simulink model "copy_final"  (R2013a)
settings: Solver=ode45  StartTime=0.0  StopTime=150  RelTol=1e-3
model workspace (MAT data in the model file):
  i = 2
undefined symbols (not defined in the file): sigbuilder_block
(part 2 of 3)

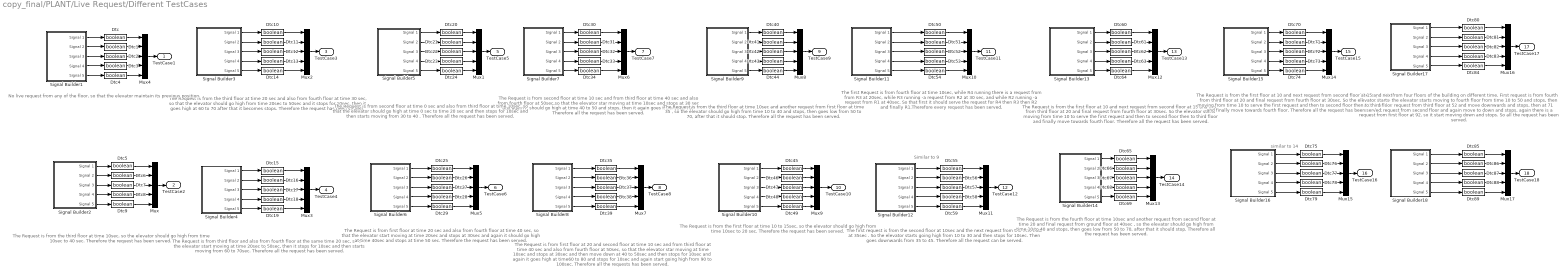
== system copy_final/PLANT/Live Request/Different TestCases ==
  note: The request is from four floors of the building on different time.
      |  First request is from fourth floor at 10, so the elevator  starts
      | moving to fourth floor from time 10 to 50 and stops, then at 50
      |  another request from third floor at 52 and move downwards
      |  and stops, then at 71 another request from second floor and
      | again move to down and stops, again there is a request from
      |  first floor at 92, so it start moving down
      | and stops. So all the request has been served.
  note: similar to 14
  note: Similar to 9
  note: The first request is from the second floor at 10sec and the next
      | request from the first floor at 35sec . So the elevator starts going
      | high from 10 to 30 and then stops for 10sec. Then goes downwards
      | from 35 to 45. Therefore all the request can be served.
  note: The Request is from third floor and also from fourth
      | floor at the same time 20 sec, so that the elevator
      | start moving at time 20sec to 50sec, then it stops
      |  for 10sec and then starts moving from 60 to 70sec.
      | Therefore all the request has been served.
  note: The Request is from the third floor at time 20 sec and
      | also from fourth floor at time 30 sec, so that the elevator
      | should go high from time 20sec to 50sec and it stops for
      | 10sec, then it goes high at 60 to 70 after that it becomes
      | stops. Therefore the request has been served.
  note: The Request is from first floor at time 20 sec and also
      |  from fourth floor at time 40 sec, so that the elevator start
      |  moving at time 20sec and stops at 30sec and again it
      | should go high at time 40sec and stops at time 50 sec.
      | Therefore the request has been served.
  note: The Request is from second floor at time 10 sec and from third
      |  floor at time 40 sec and also from fourth floor at 50sec,so that
      | the elevator star moving at time 10sec and stops at 30 sec and
      | again it should go high at time 40 to 50 and stops, then it again
      | goes from 60 to 70. Therefore all the request has been served.
  note: The Request is from first floor at 20 and second floor at time 10 sec
      |  and from third floor at time 40 sec and also from fourth floor at 50sec,
      | so that the elevator star moving at time 10sec and stops at 30sec
      | and then move down at 40 to 50sec and then stops for 10sec and
      | again it goes high at time60 to 80 and stops for 10sec and again
      |  start going high from 90 to 100sec. Therefore all the requests has
      |  been served.
  note: The Request is from the third floor at time 10sec and another
      | request from first floor at time 35 , so the elevator should go
      | high from time 10 to 40 and stops, then goes low from
      | 50 to 70, after that it should stop. Therefore all the
      |  request has been served.
  note: The Request is from the first floor at time 10 to 15sec,
      |  so the elevator should go high from time 10sec to
      | 20 sec. Therefore the request has been served.
  note: The first Request is from fourth floor at time 10sec, while R4 running there
      |  is a request from  from R3 at 20sec, while R3 running -a request from R2
      | at 30 sec, and while R2 running -a request from R1 at 40sec. So that first
      | it should serve the request for R4 then R3 then R2 and finally R1.Therefore
      |  every request has been served.
  note: The Request is from the first floor at 10 and next request from
      | second floor at 15 and next from third floor at 20 and final
      | request from fourth floor at 30sec. So the elevator starts
      | moving from time 10 to serve the first request and then to
      |  second floor  then to third floor and finally move towards
      | fourth floor. Therefore all the request has been served.
  note: No live request from any of the floor, so that
      | the elevator maintain its previous position.
  note: The Request is from the third floor at time 10sec,
      |  so the elevator should go high from time 10sec to
      | 40 sec. Therefore the request has been served.
  note: The Request is from second floor at time 0 sec and also
      |  from third floor at time 10sec, so that the elevator should
      | go high at time 0 sec  to time 20 sec and then stops for
      | 10sec and then starts moving from 30 to 40 . Therefore
      | all the request has been served.
  note: The Request is from the fourth floor at time 10sec and another
      | request from second floor at time 20 and final request from
      | ground floor at 40sec , so the elevator should go
      | high from time 10 to 40 and stops, then goes low from
      | 50 to 70, after that it should stop. Therefore all the
      |  request has been served.
  note: The Request is from the first floor at 10 and next request from
      | second floor at 15 and next from third floor at 20 and final
      | request from fourth floor at 30sec. So the elevator starts
      | moving from time 10 to serve the first request and then to
      |  second floor  then to third floor and finally move towards
      | fourth floor. Therefore all the request has been served.
  Dtc{,1..89} (90 alike) : DataTypeConversion  OutDataTypeStr=boolean
  Mux{,1..17} (18 alike) : Mux  Inputs=5
  Signal Builder1 : Subsystem  Tag=STV Subsys  LoadFcn=sigbuilder_block('load');  StartFcn=sigbuilder_block('start');  StopFcn=sigbuilder_block('stop');  ClipboardFcn=sigbuilder_block('clipboard');  mask(Sigbuilder block){}
      mask help: Simulink:masks:SigbuilderBlock_MD
      mask init:
      | if ~strcmp(get_param(bdroot(gcbh),'SimulationStatus'),'stopped') tuvar = sigbuilder_block('maskInit'); end
      settings: CopyFcn=sigbuilder_block('copy');  DeleteFcn=sigbuilder_block('delete');  ModelCloseFcn=sigbuilder_block('modelClose');  PreSaveFcn=sigbuilder_block('preSave');  PauseFcn=sigbuilder_block('pause');  ContinueFcn=sigbuilder_block('continue');  NameChangeFcn=sigbuilder_block('namechange');  OpenFcn=sigbuilder_block('open',[327.75 102.75 484.5 312.75 ]);  CloseFcn=sigbuilder_block('close');
      mask Display: plot(0, 0, 100, 100,[2, 2, 32, 32, 2], [68, 8, 8, 68, 68],[32, 2], [38, 38], [32, 19, 2],[53, 60, 44], [32, 17, 17, 2],[16, 16, 31, 31]);txt = getActiveGroup(gcbh);text(2, 100, txt,'verticalAlignment', 'top');
  Signal Builder10 : Subsystem  Tag=STV Subsys  LoadFcn=sigbuilder_block('load');  StartFcn=sigbuilder_block('start');  StopFcn=sigbuilder_block('stop');  ClipboardFcn=sigbuilder_block('clipboard');  mask(Sigbuilder block){}
      mask help: Simulink:masks:SigbuilderBlock_MD
      mask init:
      | if ~strcmp(get_param(bdroot(gcbh),'SimulationStatus'),'stopped') tuvar = sigbuilder_block('maskInit'); end
      settings: CopyFcn=sigbuilder_block('copy');  DeleteFcn=sigbuilder_block('delete');  ModelCloseFcn=sigbuilder_block('modelClose');  PreSaveFcn=sigbuilder_block('preSave');  PauseFcn=sigbuilder_block('pause');  ContinueFcn=sigbuilder_block('continue');  NameChangeFcn=sigbuilder_block('namechange');  OpenFcn=sigbuilder_block('open',[437.25 118.5 550.5 394.5 ]);  CloseFcn=sigbuilder_block('close');
      mask Display: plot(0, 0, 100, 100,[2, 2, 32, 32, 2], [68, 8, 8, 68, 68],[32, 2], [38, 38], [32, 19, 2],[53, 60, 44], [32, 17, 17, 2],[16, 16, 31, 31]);txt = getActiveGroup(gcbh);text(2, 100, txt,'verticalAlignment', 'top');
  Signal Builder11 : Subsystem  Tag=STV Subsys  LoadFcn=sigbuilder_block('load');  StartFcn=sigbuilder_block('start');  StopFcn=sigbuilder_block('stop');  ClipboardFcn=sigbuilder_block('clipboard');  mask(Sigbuilder block){}
      mask help: Simulink:masks:SigbuilderBlock_MD
      mask init:
      | if ~strcmp(get_param(bdroot(gcbh),'SimulationStatus'),'stopped') tuvar = sigbuilder_block('maskInit'); end
      settings: CopyFcn=sigbuilder_block('copy');  DeleteFcn=sigbuilder_block('delete');  ModelCloseFcn=sigbuilder_block('modelClose');  PreSaveFcn=sigbuilder_block('preSave');  PauseFcn=sigbuilder_block('pause');  ContinueFcn=sigbuilder_block('continue');  NameChangeFcn=sigbuilder_block('namechange');  OpenFcn=sigbuilder_block('open',[344.25 118.5 602.25 275.25 ]);  CloseFcn=sigbuilder_block('close');
      mask Display: plot(0, 0, 100, 100,[2, 2, 32, 32, 2], [68, 8, 8, 68, 68],[32, 2], [38, 38], [32, 19, 2],[53, 60, 44], [32, 17, 17, 2],[16, 16, 31, 31]);txt = getActiveGroup(gcbh);text(2, 100, txt,'verticalAlignment', 'top');
  Signal Builder12 : Subsystem  Tag=STV Subsys  LoadFcn=sigbuilder_block('load');  StartFcn=sigbuilder_block('start');  StopFcn=sigbuilder_block('stop');  ClipboardFcn=sigbuilder_block('clipboard');  mask(Sigbuilder block){}
      mask help: Simulink:masks:SigbuilderBlock_MD
      mask init:
      | if ~strcmp(get_param(bdroot(gcbh),'SimulationStatus'),'stopped') tuvar = sigbuilder_block('maskInit'); end
      settings: CopyFcn=sigbuilder_block('copy');  DeleteFcn=sigbuilder_block('delete');  ModelCloseFcn=sigbuilder_block('modelClose');  PreSaveFcn=sigbuilder_block('preSave');  PauseFcn=sigbuilder_block('pause');  ContinueFcn=sigbuilder_block('continue');  NameChangeFcn=sigbuilder_block('namechange');  OpenFcn=sigbuilder_block('open',[393.75 66.75 550.5 275.25 ]);  CloseFcn=sigbuilder_block('close');
      mask Display: plot(0, 0, 100, 100,[2, 2, 32, 32, 2], [68, 8, 8, 68, 68],[32, 2], [38, 38], [32, 19, 2],[53, 60, 44], [32, 17, 17, 2],[16, 16, 31, 31]);txt = getActiveGroup(gcbh);text(2, 100, txt,'verticalAlignment', 'top');
  Signal Builder13 : Subsystem  Tag=STV Subsys  LoadFcn=sigbuilder_block('load');  StartFcn=sigbuilder_block('start');  StopFcn=sigbuilder_block('stop');  ClipboardFcn=sigbuilder_block('clipboard');  mask(Sigbuilder block){}
      mask help: Simulink:masks:SigbuilderBlock_MD
      mask init:
      | if ~strcmp(get_param(bdroot(gcbh),'SimulationStatus'),'stopped') tuvar = sigbuilder_block('maskInit'); end
      settings: CopyFcn=sigbuilder_block('copy');  DeleteFcn=sigbuilder_block('delete');  ModelCloseFcn=sigbuilder_block('modelClose');  PreSaveFcn=sigbuilder_block('preSave');  PauseFcn=sigbuilder_block('pause');  ContinueFcn=sigbuilder_block('continue');  NameChangeFcn=sigbuilder_block('namechange');  OpenFcn=sigbuilder_block('open',[274.5 170.25 550.5 272.25 ]);  CloseFcn=sigbuilder_block('close');
      mask Display: plot(0, 0, 100, 100,[2, 2, 32, 32, 2], [68, 8, 8, 68, 68],[32, 2], [38, 38], [32, 19, 2],[53, 60, 44], [32, 17, 17, 2],[16, 16, 31, 31]);txt = getActiveGroup(gcbh);text(2, 100, txt,'verticalAlignment', 'top');
  Signal Builder14 : Subsystem  Tag=STV Subsys  LoadFcn=sigbuilder_block('load');  StartFcn=sigbuilder_block('start');  StopFcn=sigbuilder_block('stop');  ClipboardFcn=sigbuilder_block('clipboard');  mask(Sigbuilder block){}
      mask help: Simulink:masks:SigbuilderBlock_MD
      mask init:
      | if ~strcmp(get_param(bdroot(gcbh),'SimulationStatus'),'stopped') tuvar = sigbuilder_block('maskInit'); end
      settings: CopyFcn=sigbuilder_block('copy');  DeleteFcn=sigbuilder_block('delete');  ModelCloseFcn=sigbuilder_block('modelClose');  PreSaveFcn=sigbuilder_block('preSave');  PauseFcn=sigbuilder_block('pause');  ContinueFcn=sigbuilder_block('continue');  NameChangeFcn=sigbuilder_block('namechange');  OpenFcn=sigbuilder_block('open',[507.75 134.25 448.5 303.75 ]);  CloseFcn=sigbuilder_block('close');
      mask Display: plot(0, 0, 100, 100,[2, 2, 32, 32, 2], [68, 8, 8, 68, 68],[32, 2], [38, 38], [32, 19, 2],[53, 60, 44], [32, 17, 17, 2],[16, 16, 31, 31]);txt = getActiveGroup(gcbh);text(2, 100, txt,'verticalAlignment', 'top');
  Signal Builder15 : Subsystem  Tag=STV Subsys  LoadFcn=sigbuilder_block('load');  StartFcn=sigbuilder_block('start');  StopFcn=sigbuilder_block('stop');  ClipboardFcn=sigbuilder_block('clipboard');  mask(Sigbuilder block){}
      mask help: Simulink:masks:SigbuilderBlock_MD
      mask init:
      | if ~strcmp(get_param(bdroot(gcbh),'SimulationStatus'),'stopped') tuvar = sigbuilder_block('maskInit'); end
      settings: CopyFcn=sigbuilder_block('copy');  DeleteFcn=sigbuilder_block('delete');  ModelCloseFcn=sigbuilder_block('modelClose');  PreSaveFcn=sigbuilder_block('preSave');  PauseFcn=sigbuilder_block('pause');  ContinueFcn=sigbuilder_block('continue');  NameChangeFcn=sigbuilder_block('namechange');  OpenFcn=sigbuilder_block('open',[465.75 164.25 447 288.75 ]);  CloseFcn=sigbuilder_block('close');
      mask Display: plot(0, 0, 100, 100,[2, 2, 32, 32, 2], [68, 8, 8, 68, 68],[32, 2], [38, 38], [32, 19, 2],[53, 60, 44], [32, 17, 17, 2],[16, 16, 31, 31]);txt = getActiveGroup(gcbh);text(2, 100, txt,'verticalAlignment', 'top');
  Signal Builder16 : Subsystem  Tag=STV Subsys  LoadFcn=sigbuilder_block('load');  StartFcn=sigbuilder_block('start');  StopFcn=sigbuilder_block('stop');  ClipboardFcn=sigbuilder_block('clipboard');  mask(Sigbuilder block){}
      mask help: Simulink:masks:SigbuilderBlock_MD
      mask init:
      | if ~strcmp(get_param(bdroot(gcbh),'SimulationStatus'),'stopped') tuvar = sigbuilder_block('maskInit'); end
      settings: CopyFcn=sigbuilder_block('copy');  DeleteFcn=sigbuilder_block('delete');  ModelCloseFcn=sigbuilder_block('modelClose');  PreSaveFcn=sigbuilder_block('preSave');  PauseFcn=sigbuilder_block('pause');  ContinueFcn=sigbuilder_block('continue');  NameChangeFcn=sigbuilder_block('namechange');  OpenFcn=sigbuilder_block('open',[451.5 37.5 549 315.75 ]);  CloseFcn=sigbuilder_block('close');
      mask Display: plot(0, 0, 100, 100,[2, 2, 32, 32, 2], [68, 8, 8, 68, 68],[32, 2], [38, 38], [32, 19, 2],[53, 60, 44], [32, 17, 17, 2],[16, 16, 31, 31]);txt = getActiveGroup(gcbh);text(2, 100, txt,'verticalAlignment', 'top');
  Signal Builder17 : Subsystem  Tag=STV Subsys  LoadFcn=sigbuilder_block('load');  StartFcn=sigbuilder_block('start');  StopFcn=sigbuilder_block('stop');  ClipboardFcn=sigbuilder_block('clipboard');  mask(Sigbuilder block){}
      mask help: Simulink:masks:SigbuilderBlock_MD
      mask init:
      | if ~strcmp(get_param(bdroot(gcbh),'SimulationStatus'),'stopped') tuvar = sigbuilder_block('maskInit'); end
      settings: CopyFcn=sigbuilder_block('copy');  DeleteFcn=sigbuilder_block('delete');  ModelCloseFcn=sigbuilder_block('modelClose');  PreSaveFcn=sigbuilder_block('preSave');  PauseFcn=sigbuilder_block('pause');  ContinueFcn=sigbuilder_block('continue');  NameChangeFcn=sigbuilder_block('namechange');  OpenFcn=sigbuilder_block('open',[428.25 139.5 438.75 335.25 ]);  CloseFcn=sigbuilder_block('close');
      mask Display: plot(0, 0, 100, 100,[2, 2, 32, 32, 2], [68, 8, 8, 68, 68],[32, 2], [38, 38], [32, 19, 2],[53, 60, 44], [32, 17, 17, 2],[16, 16, 31, 31]);txt = getActiveGroup(gcbh);text(2, 100, txt,'verticalAlignment', 'top');
  Signal Builder18 : Subsystem  Tag=STV Subsys  LoadFcn=sigbuilder_block('load');  StartFcn=sigbuilder_block('start');  StopFcn=sigbuilder_block('stop');  ClipboardFcn=sigbuilder_block('clipboard');  mask(Sigbuilder block){}
      mask help: Simulink:masks:SigbuilderBlock_MD
      mask init:
      | if ~strcmp(get_param(bdroot(gcbh),'SimulationStatus'),'stopped') tuvar = sigbuilder_block('maskInit'); end
      settings: CopyFcn=sigbuilder_block('copy');  DeleteFcn=sigbuilder_block('delete');  ModelCloseFcn=sigbuilder_block('modelClose');  PreSaveFcn=sigbuilder_block('preSave');  PauseFcn=sigbuilder_block('pause');  ContinueFcn=sigbuilder_block('continue');  NameChangeFcn=sigbuilder_block('namechange');  OpenFcn=sigbuilder_block('open',[406.5 184.5 604.5 275.25 ]);  CloseFcn=sigbuilder_block('close');
      mask Display: plot(0, 0, 100, 100,[2, 2, 32, 32, 2], [68, 8, 8, 68, 68],[32, 2], [38, 38], [32, 19, 2],[53, 60, 44], [32, 17, 17, 2],[16, 16, 31, 31]);txt = getActiveGroup(gcbh);text(2, 100, txt,'verticalAlignment', 'top');
  Signal Builder2 : Subsystem  Tag=STV Subsys  LoadFcn=sigbuilder_block('load');  StartFcn=sigbuilder_block('start');  StopFcn=sigbuilder_block('stop');  ClipboardFcn=sigbuilder_block('clipboard');  mask(Sigbuilder block){}
      mask help: Simulink:masks:SigbuilderBlock_MD
      mask init:
      | if ~strcmp(get_param(bdroot(gcbh),'SimulationStatus'),'stopped') tuvar = sigbuilder_block('maskInit'); end
      settings: CopyFcn=sigbuilder_block('copy');  DeleteFcn=sigbuilder_block('delete');  ModelCloseFcn=sigbuilder_block('modelClose');  PreSaveFcn=sigbuilder_block('preSave');  PauseFcn=sigbuilder_block('pause');  ContinueFcn=sigbuilder_block('continue');  NameChangeFcn=sigbuilder_block('namechange');  OpenFcn=sigbuilder_block('open',[286.5 116.25 459.75 300.75 ]);  CloseFcn=sigbuilder_block('close');
      mask Display: plot(0, 0, 100, 100,[2, 2, 32, 32, 2], [68, 8, 8, 68, 68],[32, 2], [38, 38], [32, 19, 2],[53, 60, 44], [32, 17, 17, 2],[16, 16, 31, 31]);txt = getActiveGroup(gcbh);text(2, 100, txt,'verticalAlignment', 'top');
  Signal Builder3 : Subsystem  Tag=STV Subsys  LoadFcn=sigbuilder_block('load');  StartFcn=sigbuilder_block('start');  StopFcn=sigbuilder_block('stop');  ClipboardFcn=sigbuilder_block('clipboard');  mask(Sigbuilder block){}
      mask help: Simulink:masks:SigbuilderBlock_MD
      mask init:
      | if ~strcmp(get_param(bdroot(gcbh),'SimulationStatus'),'stopped') tuvar = sigbuilder_block('maskInit'); end
      settings: CopyFcn=sigbuilder_block('copy');  DeleteFcn=sigbuilder_block('delete');  ModelCloseFcn=sigbuilder_block('modelClose');  PreSaveFcn=sigbuilder_block('preSave');  PauseFcn=sigbuilder_block('pause');  ContinueFcn=sigbuilder_block('continue');  NameChangeFcn=sigbuilder_block('namechange');  OpenFcn=sigbuilder_block('open',[365.25 119.25 436.5 279 ]);  CloseFcn=sigbuilder_block('close');
      mask Display: plot(0, 0, 100, 100,[2, 2, 32, 32, 2], [68, 8, 8, 68, 68],[32, 2], [38, 38], [32, 19, 2],[53, 60, 44], [32, 17, 17, 2],[16, 16, 31, 31]);txt = getActiveGroup(gcbh);text(2, 100, txt,'verticalAlignment', 'top');
  Signal Builder4 : Subsystem  Tag=STV Subsys  LoadFcn=sigbuilder_block('load');  StartFcn=sigbuilder_block('start');  StopFcn=sigbuilder_block('stop');  ClipboardFcn=sigbuilder_block('clipboard');  mask(Sigbuilder block){}
      mask help: Simulink:masks:SigbuilderBlock_MD
      mask init:
      | if ~strcmp(get_param(bdroot(gcbh),'SimulationStatus'),'stopped') tuvar = sigbuilder_block('maskInit'); end
      settings: CopyFcn=sigbuilder_block('copy');  DeleteFcn=sigbuilder_block('delete');  ModelCloseFcn=sigbuilder_block('modelClose');  PreSaveFcn=sigbuilder_block('preSave');  PauseFcn=sigbuilder_block('pause');  ContinueFcn=sigbuilder_block('continue');  NameChangeFcn=sigbuilder_block('namechange');  OpenFcn=sigbuilder_block('open',[336.75 135.75 495 312.75 ]);  CloseFcn=sigbuilder_block('close');
      mask Display: plot(0, 0, 100, 100,[2, 2, 32, 32, 2], [68, 8, 8, 68, 68],[32, 2], [38, 38], [32, 19, 2],[53, 60, 44], [32, 17, 17, 2],[16, 16, 31, 31]);txt = getActiveGroup(gcbh);text(2, 100, txt,'verticalAlignment', 'top');
  Signal Builder5 : Subsystem  Tag=STV Subsys  LoadFcn=sigbuilder_block('load');  StartFcn=sigbuilder_block('start');  StopFcn=sigbuilder_block('stop');  ClipboardFcn=sigbuilder_block('clipboard');  mask(Sigbuilder block){}
      mask help: Simulink:masks:SigbuilderBlock_MD
      mask init:
      | if ~strcmp(get_param(bdroot(gcbh),'SimulationStatus'),'stopped') tuvar = sigbuilder_block('maskInit'); end
      settings: CopyFcn=sigbuilder_block('copy');  DeleteFcn=sigbuilder_block('delete');  ModelCloseFcn=sigbuilder_block('modelClose');  PreSaveFcn=sigbuilder_block('preSave');  PauseFcn=sigbuilder_block('pause');  ContinueFcn=sigbuilder_block('continue');  NameChangeFcn=sigbuilder_block('namechange');  OpenFcn=sigbuilder_block('open',[328.5 -1.5 550.5 394.5 ]);  CloseFcn=sigbuilder_block('close');
      mask Display: plot(0, 0, 100, 100,[2, 2, 32, 32, 2], [68, 8, 8, 68, 68],[32, 2], [38, 38], [32, 19, 2],[53, 60, 44], [32, 17, 17, 2],[16, 16, 31, 31]);txt = getActiveGroup(gcbh);text(2, 100, txt,'verticalAlignment', 'top');
  Signal Builder6 : Subsystem  Tag=STV Subsys  LoadFcn=sigbuilder_block('load');  StartFcn=sigbuilder_block('start');  StopFcn=sigbuilder_block('stop');  ClipboardFcn=sigbuilder_block('clipboard');  mask(Sigbuilder block){}
      mask help: Simulink:masks:SigbuilderBlock_MD
      mask init:
      | if ~strcmp(get_param(bdroot(gcbh),'SimulationStatus'),'stopped') tuvar = sigbuilder_block('maskInit'); end
      settings: CopyFcn=sigbuilder_block('copy');  DeleteFcn=sigbuilder_block('delete');  ModelCloseFcn=sigbuilder_block('modelClose');  PreSaveFcn=sigbuilder_block('preSave');  PauseFcn=sigbuilder_block('pause');  ContinueFcn=sigbuilder_block('continue');  NameChangeFcn=sigbuilder_block('namechange');  OpenFcn=sigbuilder_block('open',[91.5 55.5 550.5 394.5 ]);  CloseFcn=sigbuilder_block('close');
      mask Display: plot(0, 0, 100, 100,[2, 2, 32, 32, 2], [68, 8, 8, 68, 68],[32, 2], [38, 38], [32, 19, 2],[53, 60, 44], [32, 17, 17, 2],[16, 16, 31, 31]);txt = getActiveGroup(gcbh);text(2, 100, txt,'verticalAlignment', 'top');
  Signal Builder7 : Subsystem  Tag=STV Subsys  LoadFcn=sigbuilder_block('load');  StartFcn=sigbuilder_block('start');  StopFcn=sigbuilder_block('stop');  ClipboardFcn=sigbuilder_block('clipboard');  mask(Sigbuilder block){}
      mask help: Simulink:masks:SigbuilderBlock_MD
      mask init:
      | if ~strcmp(get_param(bdroot(gcbh),'SimulationStatus'),'stopped') tuvar = sigbuilder_block('maskInit'); end
      settings: CopyFcn=sigbuilder_block('copy');  DeleteFcn=sigbuilder_block('delete');  ModelCloseFcn=sigbuilder_block('modelClose');  PreSaveFcn=sigbuilder_block('preSave');  PauseFcn=sigbuilder_block('pause');  ContinueFcn=sigbuilder_block('continue');  NameChangeFcn=sigbuilder_block('namechange');  OpenFcn=sigbuilder_block('open',[87 91.5 512.25 357 ]);  CloseFcn=sigbuilder_block('close');
      mask Display: plot(0, 0, 100, 100,[2, 2, 32, 32, 2], [68, 8, 8, 68, 68],[32, 2], [38, 38], [32, 19, 2],[53, 60, 44], [32, 17, 17, 2],[16, 16, 31, 31]);txt = getActiveGroup(gcbh);text(2, 100, txt,'verticalAlignment', 'top');
  Signal Builder8 : Subsystem  Tag=STV Subsys  LoadFcn=sigbuilder_block('load');  StartFcn=sigbuilder_block('start');  StopFcn=sigbuilder_block('stop');  ClipboardFcn=sigbuilder_block('clipboard');  mask(Sigbuilder block){}
      mask help: Simulink:masks:SigbuilderBlock_MD
      mask init:
      | if ~strcmp(get_param(bdroot(gcbh),'SimulationStatus'),'stopped') tuvar = sigbuilder_block('maskInit'); end
      settings: CopyFcn=sigbuilder_block('copy');  DeleteFcn=sigbuilder_block('delete');  ModelCloseFcn=sigbuilder_block('modelClose');  PreSaveFcn=sigbuilder_block('preSave');  PauseFcn=sigbuilder_block('pause');  ContinueFcn=sigbuilder_block('continue');  NameChangeFcn=sigbuilder_block('namechange');  OpenFcn=sigbuilder_block('open',[269.25 168.75 480 285 ]);  CloseFcn=sigbuilder_block('close');
      mask Display: plot(0, 0, 100, 100,[2, 2, 32, 32, 2], [68, 8, 8, 68, 68],[32, 2], [38, 38], [32, 19, 2],[53, 60, 44], [32, 17, 17, 2],[16, 16, 31, 31]);txt = getActiveGroup(gcbh);text(2, 100, txt,'verticalAlignment', 'top');
  Signal Builder9 : Subsystem  Tag=STV Subsys  LoadFcn=sigbuilder_block('load');  StartFcn=sigbuilder_block('start');  StopFcn=sigbuilder_block('stop');  ClipboardFcn=sigbuilder_block('clipboard');  mask(Sigbuilder block){}
      mask help: Simulink:masks:SigbuilderBlock_MD
      mask init:
      | if ~strcmp(get_param(bdroot(gcbh),'SimulationStatus'),'stopped') tuvar = sigbuilder_block('maskInit'); end
      settings: CopyFcn=sigbuilder_block('copy');  DeleteFcn=sigbuilder_block('delete');  ModelCloseFcn=sigbuilder_block('modelClose');  PreSaveFcn=sigbuilder_block('preSave');  PauseFcn=sigbuilder_block('pause');  ContinueFcn=sigbuilder_block('continue');  NameChangeFcn=sigbuilder_block('namechange');  OpenFcn=sigbuilder_block('open',[549 141.75 414 282.75 ]);  CloseFcn=sigbuilder_block('close');
      mask Display: plot(0, 0, 100, 100,[2, 2, 32, 32, 2], [68, 8, 8, 68, 68],[32, 2], [38, 38], [32, 19, 2],[53, 60, 44], [32, 17, 17, 2],[16, 16, 31, 31]);txt = getActiveGroup(gcbh);text(2, 100, txt,'verticalAlignment', 'top');
  TestCase1 : Outport  OutDataTypeStr=boolean
  TestCase2 : Outport  Port=2  OutDataTypeStr=boolean
  TestCase3 : Outport  Port=3  OutDataTypeStr=boolean
  TestCase4 : Outport  Port=4  OutDataTypeStr=boolean
  TestCase5 : Outport  Port=5  OutDataTypeStr=boolean
  TestCase6 : Outport  Port=6  OutDataTypeStr=boolean
  TestCase7 : Outport  Port=7  OutDataTypeStr=boolean
  TestCase8 : Outport  Port=8  OutDataTypeStr=boolean
  TestCase9 : Outport  Port=9  OutDataTypeStr=boolean
  TestCase10 : Outport  Port=10  OutDataTypeStr=boolean
  TestCase11 : Outport  Port=11  OutDataTypeStr=boolean
  TestCase12 : Outport  Port=12  OutDataTypeStr=boolean
  TestCase13 : Outport  Port=13  OutDataTypeStr=boolean
  TestCase14 : Outport  Port=14  OutDataTypeStr=boolean
  TestCase15 : Outport  Port=15  OutDataTypeStr=boolean
  TestCase16 : Outport  Port=16  OutDataTypeStr=boolean
  TestCase17 : Outport  Port=17  OutDataTypeStr=boolean
  TestCase18 : Outport  Port=18  OutDataTypeStr=boolean
  wires:
  Signal Builder4/1(Signal 1) -> Dtc15/1
  Signal Builder3/4(Signal 4) -> Dtc13/1
  Mux2/1 -> TestCase3/1
  Signal Builder4/4(Signal 4) -> Dtc18/1
  Signal Builder4/3(Signal 3) -> Dtc17/1
  Mux3/1 -> TestCase4/1
  Signal Builder3/1(Signal 1) -> Dtc10/1
  Signal Builder3/2(Signal 2) -> Dtc11/1
  Signal Builder3/3(Signal 3) -> Dtc12/1
  Signal Builder4/2(Signal 2) -> Dtc16/1
  Signal Builder3/5(Signal 5) -> Dtc14/1
  Signal Builder4/5(Signal 5) -> Dtc19/1
  Dtc10/1 -> Mux2/1
  Dtc11/1 -> Mux2/2
  Dtc12/1 -> Mux2/3
  Dtc13/1 -> Mux2/4
  Dtc14/1 -> Mux2/5
  Dtc15/1 -> Mux3/1
  Dtc16/1 -> Mux3/2
  Dtc17/1 -> Mux3/3
  Dtc18/1 -> Mux3/4
  Dtc19/1 -> Mux3/5
  Signal Builder6/1(Signal 1) -> Dtc25/1
  Signal Builder6/4(Signal 4) -> Dtc28/1
  Signal Builder6/3(Signal 3) -> Dtc27/1
  Mux5/1 -> TestCase6/1
  Signal Builder6/2(Signal 2) -> Dtc26/1
  Signal Builder6/5(Signal 5) -> Dtc29/1
  Dtc25/1 -> Mux5/1
  Dtc26/1 -> Mux5/2
  Dtc27/1 -> Mux5/3
  Dtc28/1 -> Mux5/4
  Dtc29/1 -> Mux5/5
  Signal Builder7/1(Signal 1) -> Dtc30/1
  Signal Builder7/4(Signal 4) -> Dtc33/1
  Signal Builder7/3(Signal 3) -> Dtc32/1
  Mux6/1 -> TestCase7/1
  Signal Builder7/2(Signal 2) -> Dtc31/1
  Signal Builder7/5(Signal 5) -> Dtc34/1
  Dtc30/1 -> Mux6/1
  Dtc31/1 -> Mux6/2
  Dtc32/1 -> Mux6/3
  Dtc33/1 -> Mux6/4
  Dtc34/1 -> Mux6/5
  Signal Builder8/1(Signal 1) -> Dtc35/1
  Signal Builder8/4(Signal 4) -> Dtc38/1
  Signal Builder8/3(Signal 3) -> Dtc37/1
  Mux7/1 -> TestCase8/1
  Signal Builder8/2(Signal 2) -> Dtc36/1
  Signal Builder8/5(Signal 5) -> Dtc39/1
  Dtc35/1 -> Mux7/1
  Dtc36/1 -> Mux7/2
  Dtc37/1 -> Mux7/3
  Dtc38/1 -> Mux7/4
  Dtc39/1 -> Mux7/5
  Mux8/1 -> TestCase9/1
  Signal Builder9/1(Signal 1) -> Dtc40/1
  Signal Builder9/3(Signal 3) -> Dtc42/1
  Signal Builder9/5(Signal 5) -> Dtc44/1
  Signal Builder9/2(Signal 2) -> Dtc41/1
  Signal Builder9/4(Signal 4) -> Dtc43/1
  Dtc40/1 -> Mux8/1
  Dtc41/1 -> Mux8/2
  Dtc42/1 -> Mux8/3
  Dtc43/1 -> Mux8/4
  Dtc44/1 -> Mux8/5
  Mux9/1 -> TestCase10/1
  Signal Builder10/1(Signal 1) -> Dtc45/1
  Signal Builder10/3(Signal 3) -> Dtc47/1
  Signal Builder10/5(Signal 5) -> Dtc49/1
  Signal Builder10/2(Signal 2) -> Dtc46/1
  Signal Builder10/4(Signal 4) -> Dtc48/1
  Dtc45/1 -> Mux9/1
  Dtc46/1 -> Mux9/2
  Dtc47/1 -> Mux9/3
  Dtc48/1 -> Mux9/4
  Dtc49/1 -> Mux9/5
  Signal Builder11/1(Signal 1) -> Dtc50/1
  Signal Builder11/4(Signal 4) -> Dtc53/1
  Signal Builder11/3(Signal 3) -> Dtc52/1
  Mux10/1 -> TestCase11/1
  Signal Builder11/2(Signal 2) -> Dtc51/1
  Signal Builder11/5(Signal 5) -> Dtc54/1
  Dtc50/1 -> Mux10/1
  Dtc51/1 -> Mux10/2
  Dtc52/1 -> Mux10/3
  Dtc53/1 -> Mux10/4
  Dtc54/1 -> Mux10/5
  Signal Builder12/1(Signal 1) -> Dtc55/1
  Signal Builder12/4(Signal 4) -> Dtc58/1
  Signal Builder12/3(Signal 3) -> Dtc57/1
  Mux11/1 -> TestCase12/1
  Signal Builder12/2(Signal 2) -> Dtc56/1
  Dtc55/1 -> Mux11/1
  Dtc56/1 -> Mux11/2
  Dtc57/1 -> Mux11/3
  Dtc58/1 -> Mux11/4
  Dtc59/1 -> Mux11/5
  Signal Builder12/5(Signal 5) -> Dtc59/1
  Signal Builder13/4(Signal 4) -> Dtc63/1
  Mux12/1 -> TestCase13/1
  Signal Builder13/1(Signal 1) -> Dtc60/1
  Signal Builder13/2(Signal 2) -> Dtc61/1
  Signal Builder13/3(Signal 3) -> Dtc62/1
  Signal Builder13/5(Signal 5) -> Dtc64/1
  Dtc60/1 -> Mux12/1
  Dtc61/1 -> Mux12/2
  Dtc62/1 -> Mux12/3
  Dtc63/1 -> Mux12/4
  Dtc64/1 -> Mux12/5
  Mux4/1 -> TestCase1/1
  Dtc/1 -> Mux4/1
  Dtc1/1 -> Mux4/2
  Dtc2/1 -> Mux4/3
  Dtc3/1 -> Mux4/4
  Dtc4/1 -> Mux4/5
  Mux/1 -> TestCase2/1
  Signal Builder2/1(Signal 1) -> Dtc5/1
  Signal Builder2/3(Signal 3) -> Dtc7/1
  Signal Builder2/5(Signal 5) -> Dtc9/1
  Signal Builder2/2(Signal 2) -> Dtc6/1
  Signal Builder2/4(Signal 4) -> Dtc8/1
  Dtc5/1 -> Mux/1
  Dtc6/1 -> Mux/2
  Dtc7/1 -> Mux/3
  Dtc8/1 -> Mux/4
  Dtc9/1 -> Mux/5
  Mux1/1 -> TestCase5/1
  Signal Builder5/4(Signal 4) -> Dtc23/1
  Signal Builder5/5(Signal 5) -> Dtc24/1
  Signal Builder5/3(Signal 3) -> Dtc22/1
  Signal Builder5/2(Signal 2) -> Dtc21/1
  Dtc21/1 -> Mux1/2
  Dtc22/1 -> Mux1/3
  Dtc23/1 -> Mux1/4
  Dtc24/1 -> Mux1/5
  Signal Builder5/1(Signal 1) -> Dtc20/1
  Dtc20/1 -> Mux1/1
  Signal Builder1/1(Signal 1) -> Dtc/1
  Signal Builder1/2(Signal 2) -> Dtc1/1
  Signal Builder1/3(Signal 3) -> Dtc2/1
  Signal Builder1/4(Signal 4) -> Dtc3/1
  Signal Builder1/5(Signal 5) -> Dtc4/1
  Mux13/1 -> TestCase14/1
  Signal Builder14/1(Signal 1) -> Dtc65/1
  Signal Builder14/3(Signal 3) -> Dtc67/1
  Signal Builder14/2(Signal 2) -> Dtc66/1
  Signal Builder14/4(Signal 4) -> Dtc68/1
  Dtc65/1 -> Mux13/1
  Dtc66/1 -> Mux13/2
  Dtc67/1 -> Mux13/3
  Dtc68/1 -> Mux13/4
  Dtc69/1 -> Mux13/5
  Signal Builder14/5(Signal 5) -> Dtc69/1
  Signal Builder15/4(Signal 4) -> Dtc73/1
  Mux14/1 -> TestCase15/1
  Signal Builder15/1(Signal 1) -> Dtc70/1
  Signal Builder15/2(Signal 2) -> Dtc71/1
  Signal Builder15/3(Signal 3) -> Dtc72/1
  Signal Builder15/5(Signal 5) -> Dtc74/1
  Dtc70/1 -> Mux14/1
  Dtc71/1 -> Mux14/2
  Dtc72/1 -> Mux14/3
  Dtc73/1 -> Mux14/4
  Dtc74/1 -> Mux14/5
  Signal Builder16/4(Signal 4) -> Dtc78/1
  Mux15/1 -> TestCase16/1
  Signal Builder16/1(Signal 1) -> Dtc75/1
  Signal Builder16/2(Signal 2) -> Dtc76/1
  Signal Builder16/3(Signal 3) -> Dtc77/1
  Signal Builder16/5(Signal 5) -> Dtc79/1
  Dtc75/1 -> Mux15/1
  Dtc76/1 -> Mux15/2
  Dtc77/1 -> Mux15/3
  Dtc78/1 -> Mux15/4
  Dtc79/1 -> Mux15/5
  Signal Builder17/1(Signal 1) -> Dtc80/1
  Signal Builder17/4(Signal 4) -> Dtc83/1
  Signal Builder17/3(Signal 3) -> Dtc82/1
  Mux16/1 -> TestCase17/1
  Signal Builder17/2(Signal 2) -> Dtc81/1
  Signal Builder17/5(Signal 5) -> Dtc84/1
  Dtc80/1 -> Mux16/1
  Dtc81/1 -> Mux16/2
  Dtc82/1 -> Mux16/3
  Dtc83/1 -> Mux16/4
  Dtc84/1 -> Mux16/5
  Signal Builder18/1(Signal 1) -> Dtc85/1
  Signal Builder18/4(Signal 4) -> Dtc88/1
  Signal Builder18/3(Signal 3) -> Dtc87/1
  Mux17/1 -> TestCase18/1
  Signal Builder18/2(Signal 2) -> Dtc86/1
  Signal Builder18/5(Signal 5) -> Dtc89/1
  Dtc85/1 -> Mux17/1
  Dtc86/1 -> Mux17/2
  Dtc87/1 -> Mux17/3
  Dtc88/1 -> Mux17/4
  Dtc89/1 -> Mux17/5

== system copy_final/PLANT/Position Id/Subsystem ==
  position : Inport  OutDataTypeStr=int32
  Constant : Constant  Value=40  OutDataTypeStr=int32
  Data Type Conversion : DataTypeConversion  OutDataTypeStr=boolean
  Relational Operator1 : RelationalOperator  Operator===  OutDataTypeStr=boolean
  "p4 " : Outport  OutDataTypeStr=boolean
  wires:
  Relational Operator1/1 -> Data Type Conversion/1
  Data Type Conversion/1 -> "p4 "/1
  Constant/1 -> Relational Operator1/2
  position/1 -> Relational Operator1/1

== system copy_final/PLANT/Position Id/Subsystem1 ==
  position : Inport  OutDataTypeStr=int32
  Constant : Constant  Value=30  OutDataTypeStr=int32
  Data Type Conversion : DataTypeConversion  OutDataTypeStr=boolean
  Relational Operator1 : RelationalOperator  Operator===  OutDataTypeStr=boolean
  "p3 " : Outport  OutDataTypeStr=boolean
  wires:
  position/1 -> Relational Operator1/1
  Relational Operator1/1 -> Data Type Conversion/1
  Constant/1 -> Relational Operator1/2
  Data Type Conversion/1 -> "p3 "/1

== system copy_final/PLANT/Position Id/Subsystem2 ==
  position : Inport  OutDataTypeStr=int32
  Constant : Constant  Value=20  OutDataTypeStr=int32
  Data Type Conversion : DataTypeConversion  OutDataTypeStr=boolean
  Relational Operator1 : RelationalOperator  Operator===  OutDataTypeStr=boolean
  "p2 " : Outport  OutDataTypeStr=boolean
  wires:
  position/1 -> Relational Operator1/1
  Relational Operator1/1 -> Data Type Conversion/1
  Data Type Conversion/1 -> "p2 "/1
  Constant/1 -> Relational Operator1/2

== system copy_final/PLANT/Position Id/Subsystem3 ==
  position : Inport  OutDataTypeStr=int32
  Constant : Constant  Value=10  OutDataTypeStr=int32
  Data Type Conversion : DataTypeConversion  OutDataTypeStr=boolean
  Relational Operator1 : RelationalOperator  Operator===  OutDataTypeStr=boolean
  "p1 " : Outport  OutDataTypeStr=boolean
  wires:
  position/1 -> Relational Operator1/1
  Relational Operator1/1 -> Data Type Conversion/1
  Data Type Conversion/1 -> "p1 "/1
  Constant/1 -> Relational Operator1/2

== system copy_final/PLANT/Position Id/Subsystem4 ==
  position : Inport  OutDataTypeStr=int32
  Constant : Constant  Value=0  OutDataTypeStr=int32
  Data Type Conversion : DataTypeConversion  OutDataTypeStr=boolean
  Relational Operator1 : RelationalOperator  Operator===  OutDataTypeStr=boolean
  "p0 " : Outport  OutDataTypeStr=boolean
  wires:
  position/1 -> Relational Operator1/1
  Relational Operator1/1 -> Data Type Conversion/1
  Data Type Conversion/1 -> "p0 "/1
  Constant/1 -> Relational Operator1/2

== system copy_final/ELEVATOR/DIRECTION/LiveRequest(T//F)/Subsystem ==
  Absolute Value : Inport  OutDataTypeStr=int32
  R4out : Inport  Port=2  OutDataTypeStr=boolean
  Constant : Constant  Value=100  OutDataTypeStr=int32
  Multiport Switch2 : MultiPortSwitch  DataPortOrder=Zero-based contiguous  Inputs=2  DiagnosticForDefault=None  OutDataTypeStr=int32
  R4outt : Outport  OutDataTypeStr=int32
  wires:
  Multiport Switch2/1 -> R4outt/1
  R4out/1 -> Multiport Switch2/1
  Constant/1 -> Multiport Switch2/2
  Absolute Value/1 -> Multiport Switch2/3

== system copy_final/ELEVATOR/DIRECTION/LiveRequest(T//F)/Subsystem1 ==
  Absolute Value : Inport  OutDataTypeStr=int32
  R3out : Inport  Port=2  OutDataTypeStr=boolean
  Constant : Constant  Value=100  OutDataTypeStr=int32
  Multiport Switch : MultiPortSwitch  DataPortOrder=Zero-based contiguous  Inputs=2  DiagnosticForDefault=None  OutDataTypeStr=int32
  R3outt : Outport  OutDataTypeStr=int32
  wires:
  Multiport Switch/1 -> R3outt/1
  R3out/1 -> Multiport Switch/1
  Constant/1 -> Multiport Switch/2
  Absolute Value/1 -> Multiport Switch/3

== system copy_final/ELEVATOR/DIRECTION/LiveRequest(T//F)/Subsystem2 ==
  Absolute Value : Inport  OutDataTypeStr=int32
  R2out : Inport  Port=2  OutDataTypeStr=boolean
  Constant : Constant  Value=100  OutDataTypeStr=int32
  Multiport Switch : MultiPortSwitch  DataPortOrder=Zero-based contiguous  Inputs=2  DiagnosticForDefault=None  OutDataTypeStr=int32
  R2outt : Outport  OutDataTypeStr=int32
  wires:
  Multiport Switch/1 -> R2outt/1
  R2out/1 -> Multiport Switch/1
  Constant/1 -> Multiport Switch/2
  Absolute Value/1 -> Multiport Switch/3

== system copy_final/ELEVATOR/DIRECTION/LiveRequest(T//F)/Subsystem3 ==
  Absolute Value : Inport  OutDataTypeStr=int32
  R1out : Inport  Port=2  OutDataTypeStr=boolean
  Constant : Constant  Value=100  OutDataTypeStr=int32
  Multiport Switch : MultiPortSwitch  DataPortOrder=Zero-based contiguous  Inputs=2  DiagnosticForDefault=None  OutDataTypeStr=int32
  R1outt : Outport  OutDataTypeStr=int32
  wires:
  Multiport Switch/1 -> R1outt/1
  R1out/1 -> Multiport Switch/1
  Constant/1 -> Multiport Switch/2
  Absolute Value/1 -> Multiport Switch/3

== system copy_final/ELEVATOR/DIRECTION/LiveRequest(T//F)/Subsystem4 ==
  Absolute Value : Inport  OutDataTypeStr=int32
  R0out : Inport  Port=2  OutDataTypeStr=boolean
  Constant : Constant  Value=100  OutDataTypeStr=int32
  Multiport Switch : MultiPortSwitch  DataPortOrder=Zero-based contiguous  Inputs=2  DiagnosticForDefault=None  OutDataTypeStr=int32
  R0outt : Outport  OutDataTypeStr=int32
  wires:
  Multiport Switch/1 -> R0outt/1
  R0out/1 -> Multiport Switch/1
  Constant/1 -> Multiport Switch/2
  Absolute Value/1 -> Multiport Switch/3

== system copy_final/ELEVATOR/DIRECTION/Requested Floor/Subsystem ==
  R4outt : Inport  OutDataTypeStr=int32
  MinMax : Inport  Port=2  OutDataTypeStr=int32
  Complex to Real-Imag : ComplexToRealImag
  Constant : Constant  Value=4  OutDataTypeStr=int32
  Constant1 : Constant  Value=100  OutDataTypeStr=int32
  Multiport Switch : MultiPortSwitch  DataPortOrder=Zero-based contiguous  Inputs=2  DiagnosticForDefault=None  OutDataTypeStr=int32
  Relational Operator : RelationalOperator  Operator===  OutDataTypeStr=boolean
  F4Out : Outport  OutDataTypeStr=int32
  wires:
  R4outt/1 -> Relational Operator/1
  MinMax/1 -> Relational Operator/2
  Multiport Switch/1 -> F4Out/1
  Constant/1 -> Complex to Real-Imag/1
  Relational Operator/1 -> Multiport Switch/1
  Constant1/1 -> Multiport Switch/2
  Complex to Real-Imag/1 -> Multiport Switch/3

== system copy_final/ELEVATOR/DIRECTION/Requested Floor/Subsystem1 ==
  R3outt : Inport  OutDataTypeStr=int32
  MinMax : Inport  Port=2  OutDataTypeStr=int32
  Complex to Real-Imag : ComplexToRealImag
  Constant : Constant  Value=3  OutDataTypeStr=int32
  Constant1 : Constant  Value=100  OutDataTypeStr=int32
  Multiport Switch : MultiPortSwitch  DataPortOrder=Zero-based contiguous  Inputs=2  DiagnosticForDefault=None  OutDataTypeStr=int32
  Relational Operator : RelationalOperator  Operator===  OutDataTypeStr=boolean
  F3Out : Outport  OutDataTypeStr=int32
  wires:
  R3outt/1 -> Relational Operator/1
  MinMax/1 -> Relational Operator/2
  Multiport Switch/1 -> F3Out/1
  Constant/1 -> Complex to Real-Imag/1
  Relational Operator/1 -> Multiport Switch/1
  Constant1/1 -> Multiport Switch/2
  Complex to Real-Imag/1 -> Multiport Switch/3

== system copy_final/ELEVATOR/DIRECTION/Requested Floor/Subsystem2 ==
  R2outt : Inport  OutDataTypeStr=int32
  MinMax : Inport  Port=2  OutDataTypeStr=int32
  Complex to Real-Imag : ComplexToRealImag
  Constant : Constant  Value=2  OutDataTypeStr=int32
  Constant1 : Constant  Value=100  OutDataTypeStr=int32
  Multiport Switch : MultiPortSwitch  DataPortOrder=Zero-based contiguous  Inputs=2  DiagnosticForDefault=None  OutDataTypeStr=int32
  Relational Operator : RelationalOperator  Operator===  OutDataTypeStr=boolean
  F2Out : Outport  OutDataTypeStr=int32
  wires:
  R2outt/1 -> Relational Operator/1
  MinMax/1 -> Relational Operator/2
  Multiport Switch/1 -> F2Out/1
  Constant/1 -> Complex to Real-Imag/1
  Relational Operator/1 -> Multiport Switch/1
  Constant1/1 -> Multiport Switch/2
  Complex to Real-Imag/1 -> Multiport Switch/3

== system copy_final/ELEVATOR/DIRECTION/Requested Floor/Subsystem3 ==
  R1outt : Inport  OutDataTypeStr=int32
  MinMax : Inport  Port=2  OutDataTypeStr=int32
  Complex to Real-Imag : ComplexToRealImag
  Constant : Constant  OutDataTypeStr=int32
  Constant1 : Constant  Value=100  OutDataTypeStr=int32
  Multiport Switch : MultiPortSwitch  DataPortOrder=Zero-based contiguous  Inputs=2  DiagnosticForDefault=None  OutDataTypeStr=int32
  Relational Operator : RelationalOperator  Operator===  OutDataTypeStr=boolean
  F1Out : Outport  OutDataTypeStr=int32
  wires:
  R1outt/1 -> Relational Operator/1
  MinMax/1 -> Relational Operator/2
  Multiport Switch/1 -> F1Out/1
  Constant/1 -> Complex to Real-Imag/1
  Relational Operator/1 -> Multiport Switch/1
  Constant1/1 -> Multiport Switch/2
  Complex to Real-Imag/1 -> Multiport Switch/3

== system copy_final/ELEVATOR/DIRECTION/Requested Floor/Subsystem4 ==
  R0outt : Inport  OutDataTypeStr=int32
  MinMax : Inport  Port=2  OutDataTypeStr=int32
  Complex to Real-Imag : ComplexToRealImag
  Constant : Constant  Value=0  OutDataTypeStr=int32
  Constant1 : Constant  Value=100  OutDataTypeStr=int32
  Multiport Switch : MultiPortSwitch  DataPortOrder=Zero-based contiguous  Inputs=2  DiagnosticForDefault=None  OutDataTypeStr=int32
  Relational Operator : RelationalOperator  Operator===  OutDataTypeStr=boolean
  F0Out : Outport  OutDataTypeStr=int32
  wires:
  R0outt/1 -> Relational Operator/1
  MinMax/1 -> Relational Operator/2
  Multiport Switch/1 -> F0Out/1
  Constant/1 -> Complex to Real-Imag/1
  Relational Operator/1 -> Multiport Switch/1
  Constant1/1 -> Multiport Switch/2
  Complex to Real-Imag/1 -> Multiport Switch/3

== system copy_final/PLANT/Live Request/Different TestCases/Signal Builder1 ==
  Demux : Demux  Tag=STV Demux  Outputs=5
  FromWs : FromWorkspace  Tag=STV FromWs  VariableName=tuvar  SampleTime=0
      SigBuilderData=|
      | common.afterFinalStr = 'Extrapolate'
      | common.sampleTime = 0
      | dataSet.timeRange = [0 50]
      | dataSet.name = 'Group 1'
      | sbobj.Groups.Name = 'Group 1'
      | sbobj.Groups.Signals(1).Name = 'Signal 1'
      | sbobj.Groups.Signals(1).XData = [0 30 31 50]
      | sbobj.Groups.Signals(1).YData = [0 0 0 0]
      | sbobj.Groups.Signals(2).Name = 'Signal 2'
      | sbobj.Groups.Signals(2).XData = [0 20 21 50]
      | sbobj.Groups.Signals(2).YData = [0 0 0 0]
      | sbobj.Groups.Signals(3).Name = 'Signal 3'
      | sbobj.Groups.Signals(3).XData = [0 21 30 50]
      | sbobj.Groups.Signals(3).YData = [0 0 0 0]
      | sbobj.Groups.Signals(4).Name = 'Signal 4'
      | sbobj.Groups.Signals(4).XData = [0 10 11 50]
      | sbobj.Groups.Signals(4).YData = [0 0 0 0]
      | sbobj.Groups.Signals(5).Name = 'Signal 5'
      | sbobj.Groups.Signals(5).XData = [0 40 50]
      | sbobj.Groups.Signals(5).YData = [0 0 0]
      | sbobj.Groups.TimeRange = [0 50]
  Signal 1 : Outport  Tag=STV Outport
  Signal 2 : Outport  Tag=STV Outport  Port=2
  Signal 3 : Outport  Tag=STV Outport  Port=3
  Signal 4 : Outport  Tag=STV Outport  Port=4
  Signal 5 : Outport  Tag=STV Outport  Port=5
  wires:
  Demux/1 -> Signal 1/1
  FromWs/1 -> Demux/1
  Demux/2 -> Signal 2/1
  Demux/3 -> Signal 3/1
  Demux/4 -> Signal 4/1
  Demux/5 -> Signal 5/1

== system copy_final/PLANT/Live Request/Different TestCases/Signal Builder10 ==
  Demux : Demux  Tag=STV Demux  Outputs=5
  FromWs : FromWorkspace  Tag=STV FromWs  VariableName=tuvar  SampleTime=0
      SigBuilderData=|
      | common.afterFinalStr = 'Extrapolate'
      | common.sampleTime = 0
      | dataSet.timeRange = [0 50]
      | dataSet.name = 'Group 1'
      | sbobj.Groups.Name = 'Group 1'
      | sbobj.Groups.Signals(1).Name = 'Signal 1'
      | sbobj.Groups.Signals(1).XData = [0 4 6 50]
      | sbobj.Groups.Signals(1).YData = [0 0 0 0]
      | sbobj.Groups.Signals(2).Name = 'Signal 2'
      | sbobj.Groups.Signals(2).XData = [0 10 11 50]
      | sbobj.Groups.Signals(2).YData = [0 0 0 0]
      | sbobj.Groups.Signals(3).Name = 'Signal 3'
      | sbobj.Groups.Signals(3).XData = [0 21 30 50]
      | sbobj.Groups.Signals(3).YData = [0 0 0 0]
      | sbobj.Groups.Signals(4).Name = 'Signal 4'
      | sbobj.Groups.Signals(4).XData = [0 10 10 15 15 50]
      | sbobj.Groups.Signals(4).YData = [0 0 1 1 0 0]
      | sbobj.Groups.Signals(5).Name = 'Signal 5'
      | sbobj.Groups.Signals(5).XData = [0 40 50]
      | sbobj.Groups.Signals(5).YData = [0 0 0]
      | sbobj.Groups.TimeRange = [0 50]
  Signal 1 : Outport  Tag=STV Outport
  Signal 2 : Outport  Tag=STV Outport  Port=2
  Signal 3 : Outport  Tag=STV Outport  Port=3
  Signal 4 : Outport  Tag=STV Outport  Port=4
  Signal 5 : Outport  Tag=STV Outport  Port=5
  wires:
  Demux/1 -> Signal 1/1
  FromWs/1 -> Demux/1
  Demux/2 -> Signal 2/1
  Demux/3 -> Signal 3/1
  Demux/4 -> Signal 4/1
  Demux/5 -> Signal 5/1

== system copy_final/PLANT/Live Request/Different TestCases/Signal Builder11 ==
  Demux : Demux  Tag=STV Demux  Outputs=5
  FromWs : FromWorkspace  Tag=STV FromWs  VariableName=tuvar  SampleTime=0
      SigBuilderData=|
      | common.afterFinalStr = 'Extrapolate'
      | common.sampleTime = 0
      | dataSet.timeRange = [0 100]
      | dataSet.name = 'Group 1'
      | sbobj.Groups.Name = 'Group 1'
      | sbobj.Groups.Signals(1).Name = 'Signal 1'
      | sbobj.Groups.Signals(1).XData = [0 10 10 11 11 100]
      | sbobj.Groups.Signals(1).YData = [0 0 1 1 0 0]
      | sbobj.Groups.Signals(2).Name = 'Signal 2'
      | sbobj.Groups.Signals(2).XData = [0 20.1 20.1 21 21 100]
      | sbobj.Groups.Signals(2).YData = [0 0 1 1 0 0]
      | sbobj.Groups.Signals(3).Name = 'Signal 3'
      | sbobj.Groups.Signals(3).XData = [0 30 30 31 31 100]
      | sbobj.Groups.Signals(3).YData = [0 0 1 1 0 0]
      | sbobj.Groups.Signals(4).Name = 'Signal 4'
      | sbobj.Groups.Signals(4).XData = [0 40 40 41 41 100]
      | sbobj.Groups.Signals(4).YData = [0 0 1 1 0 0]
      | sbobj.Groups.Signals(5).Name = 'Signal 5'
      | sbobj.Groups.Signals(5).XData = [0 40 100]
      | sbobj.Groups.Signals(5).YData = [0 0 0]
      | sbobj.Groups.TimeRange = [0 100]
  Signal 1 : Outport  Tag=STV Outport
  Signal 2 : Outport  Tag=STV Outport  Port=2
  Signal 3 : Outport  Tag=STV Outport  Port=3
  Signal 4 : Outport  Tag=STV Outport  Port=4
  Signal 5 : Outport  Tag=STV Outport  Port=5
  wires:
  Demux/1 -> Signal 1/1
  FromWs/1 -> Demux/1
  Demux/2 -> Signal 2/1
  Demux/3 -> Signal 3/1
  Demux/4 -> Signal 4/1
  Demux/5 -> Signal 5/1

== system copy_final/PLANT/Live Request/Different TestCases/Signal Builder12 ==
  Demux : Demux  Tag=STV Demux  Outputs=5
  FromWs : FromWorkspace  Tag=STV FromWs  VariableName=tuvar  SampleTime=0
      SigBuilderData=|
      | common.afterFinalStr = 'Extrapolate'
      | common.sampleTime = 0
      | dataSet.timeRange = [0 50]
      | dataSet.name = 'Group 1'
      | sbobj.Groups.Name = 'Group 1'
      | sbobj.Groups.Signals(1).Name = 'Signal 1'
      | sbobj.Groups.Signals(1).XData = [0 10 11 50]
      | sbobj.Groups.Signals(1).YData = [0 0 0 0]
      | sbobj.Groups.Signals(2).Name = 'Signal 2'
      | sbobj.Groups.Signals(2).XData = [0 20.1 21 50]
      | sbobj.Groups.Signals(2).YData = [0 0 0 0]
      | sbobj.Groups.Signals(3).Name = 'Signal 3'
      | sbobj.Groups.Signals(3).XData = [0 10 10 11 11 50]
      | sbobj.Groups.Signals(3).YData = [0 0 1 1 0 0]
      | sbobj.Groups.Signals(4).Name = 'Signal 4'
      | sbobj.Groups.Signals(4).XData = [0 31 31 32 32 50]
      | sbobj.Groups.Signals(4).YData = [0 0 1 1 0 0]
      | sbobj.Groups.Signals(5).Name = 'Signal 5'
      | sbobj.Groups.Signals(5).XData = [0 35 36 50]
      | sbobj.Groups.Signals(5).YData = [0 0 0 0]
      | sbobj.Groups.TimeRange = [0 50]
  Signal 1 : Outport  Tag=STV Outport
  Signal 2 : Outport  Tag=STV Outport  Port=2
  Signal 3 : Outport  Tag=STV Outport  Port=3
  Signal 4 : Outport  Tag=STV Outport  Port=4
  Signal 5 : Outport  Tag=STV Outport  Port=5
  wires:
  Demux/1 -> Signal 1/1
  FromWs/1 -> Demux/1
  Demux/2 -> Signal 2/1
  Demux/3 -> Signal 3/1
  Demux/4 -> Signal 4/1
  Demux/5 -> Signal 5/1

== system copy_final/PLANT/Live Request/Different TestCases/Signal Builder13 ==
  Demux : Demux  Tag=STV Demux  Outputs=5
  FromWs : FromWorkspace  Tag=STV FromWs  VariableName=tuvar  SampleTime=0
      SigBuilderData=|
      | common.afterFinalStr = 'Extrapolate'
      | common.sampleTime = 0
      | dataSet.timeRange = [0 50]
      | dataSet.name = 'Group 1'
      | sbobj.Groups.Name = 'Group 1'
      | sbobj.Groups.Signals(1).Name = 'Signal 1'
      | sbobj.Groups.Signals(1).XData = [0 30 30 31 31 50]
      | sbobj.Groups.Signals(1).YData = [0 0 1 1 0 0]
      | sbobj.Groups.Signals(2).Name = 'Signal 2'
      | sbobj.Groups.Signals(2).XData = [0 20 20 21 21 50]
      | sbobj.Groups.Signals(2).YData = [0 0 1 1 0 0]
      | sbobj.Groups.Signals(3).Name = 'Signal 3'
      | sbobj.Groups.Signals(3).XData = [0 15 15 16 16 50]
      | sbobj.Groups.Signals(3).YData = [0 0 1 1 0 0]
      | sbobj.Groups.Signals(4).Name = 'Signal 4'
      | sbobj.Groups.Signals(4).XData = [0 10 10 11 11 50]
      | sbobj.Groups.Signals(4).YData = [0 0 0.95 0.95 0 0]
      | sbobj.Groups.Signals(5).Name = 'Signal 5'
      | sbobj.Groups.Signals(5).XData = [0 40 50]
      | sbobj.Groups.Signals(5).YData = [0 0 0]
      | sbobj.Groups.TimeRange = [0 50]
  Signal 1 : Outport  Tag=STV Outport
  Signal 2 : Outport  Tag=STV Outport  Port=2
  Signal 3 : Outport  Tag=STV Outport  Port=3
  Signal 4 : Outport  Tag=STV Outport  Port=4
  Signal 5 : Outport  Tag=STV Outport  Port=5
  wires:
  Demux/1 -> Signal 1/1
  FromWs/1 -> Demux/1
  Demux/2 -> Signal 2/1
  Demux/3 -> Signal 3/1
  Demux/4 -> Signal 4/1
  Demux/5 -> Signal 5/1

== system copy_final/PLANT/Live Request/Different TestCases/Signal Builder14 ==
  Demux : Demux  Tag=STV Demux  Outputs=5
  FromWs : FromWorkspace  Tag=STV FromWs  VariableName=tuvar  SampleTime=0
      SigBuilderData=|
      | common.afterFinalStr = 'Extrapolate'
      | common.sampleTime = 0
      | dataSet.timeRange = [0 50]
      | dataSet.name = 'Group 1'
      | sbobj.Groups.Name = 'Group 1'
      | sbobj.Groups.Signals(1).Name = 'Signal 1'
      | sbobj.Groups.Signals(1).XData = [0 10 10 11 11 50]
      | sbobj.Groups.Signals(1).YData = [0 0 1 1 0 0]
      | sbobj.Groups.Signals(2).Name = 'Signal 2'
      | sbobj.Groups.Signals(2).XData = [0 10 11 50]
      | sbobj.Groups.Signals(2).YData = [0 0 0 0]
      | sbobj.Groups.Signals(3).Name = 'Signal 3'
      | sbobj.Groups.Signals(3).XData = [0 20 20 21 21 50]
      | sbobj.Groups.Signals(3).YData = [0 0 1 1 0 0]
      | sbobj.Groups.Signals(4).Name = 'Signal 4'
      | sbobj.Groups.Signals(4).XData = [0 20.05 36 50]
      | sbobj.Groups.Signals(4).YData = [0 0 0 0]
      | sbobj.Groups.Signals(5).Name = 'Signal 5'
      | sbobj.Groups.Signals(5).XData = [0 40 41 50]
      | sbobj.Groups.Signals(5).YData = [0 0 0 0]
      | sbobj.Groups.TimeRange = [0 50]
  Signal 1 : Outport  Tag=STV Outport
  Signal 2 : Outport  Tag=STV Outport  Port=2
  Signal 3 : Outport  Tag=STV Outport  Port=3
  Signal 4 : Outport  Tag=STV Outport  Port=4
  Signal 5 : Outport  Tag=STV Outport  Port=5
  wires:
  Demux/1 -> Signal 1/1
  FromWs/1 -> Demux/1
  Demux/2 -> Signal 2/1
  Demux/3 -> Signal 3/1
  Demux/4 -> Signal 4/1
  Demux/5 -> Signal 5/1

== system copy_final/PLANT/Live Request/Different TestCases/Signal Builder15 ==
  Demux : Demux  Tag=STV Demux  Outputs=5
  FromWs : FromWorkspace  Tag=STV FromWs  VariableName=tuvar  SampleTime=0
      SigBuilderData=|
      | common.afterFinalStr = 'Extrapolate'
      | common.sampleTime = 0
      | dataSet.timeRange = [0 50]
      | dataSet.name = 'Group 1'
      | sbobj.Groups.Name = 'Group 1'
      | sbobj.Groups.Signals(1).Name = 'Signal 1'
      | sbobj.Groups.Signals(1).XData = [0 30 30 31 31 50]
      | sbobj.Groups.Signals(1).YData = [0 0 1 1 0 0]
      | sbobj.Groups.Signals(2).Name = 'Signal 2'
      | sbobj.Groups.Signals(2).XData = [0 20 20 21 21 50]
      | sbobj.Groups.Signals(2).YData = [0 0 1 1 0 0]
      | sbobj.Groups.Signals(3).Name = 'Signal 3'
      | sbobj.Groups.Signals(3).XData = [0 15 15 16 16 50]
      | sbobj.Groups.Signals(3).YData = [0 0 1 1 0 0]
      | sbobj.Groups.Signals(4).Name = 'Signal 4'
      | sbobj.Groups.Signals(4).XData = [0 35 35 36 36 50]
      | sbobj.Groups.Signals(4).YData = [0 0 1 1 0 0]
      | sbobj.Groups.Signals(5).Name = 'Signal 5'
      | sbobj.Groups.Signals(5).XData = [0 40 50]
      | sbobj.Groups.Signals(5).YData = [0 0 0]
      | sbobj.Groups.TimeRange = [0 50]
  Signal 1 : Outport  Tag=STV Outport
  Signal 2 : Outport  Tag=STV Outport  Port=2
  Signal 3 : Outport  Tag=STV Outport  Port=3
  Signal 4 : Outport  Tag=STV Outport  Port=4
  Signal 5 : Outport  Tag=STV Outport  Port=5
  wires:
  Demux/1 -> Signal 1/1
  FromWs/1 -> Demux/1
  Demux/2 -> Signal 2/1
  Demux/3 -> Signal 3/1
  Demux/4 -> Signal 4/1
  Demux/5 -> Signal 5/1

== system copy_final/PLANT/Live Request/Different TestCases/Signal Builder16 ==
  Demux : Demux  Tag=STV Demux  Outputs=5
  FromWs : FromWorkspace  Tag=STV FromWs  VariableName=tuvar  SampleTime=0
      SigBuilderData=|
      | common.afterFinalStr = 'Extrapolate'
      | common.sampleTime = 0
      | dataSet.timeRange = [0 50]
      | dataSet.name = 'Group 1'
      | sbobj.Groups.Name = 'Group 1'
      | sbobj.Groups.Signals(1).Name = 'Signal 1'
      | sbobj.Groups.Signals(1).XData = [0 10 10 11 11 50]
      | sbobj.Groups.Signals(1).YData = [0 0 1 1 0 0]
      | sbobj.Groups.Signals(2).Name = 'Signal 2'
      | sbobj.Groups.Signals(2).XData = [0 20 21 50]
      | sbobj.Groups.Signals(2).YData = [0 0 0 0]
      | sbobj.Groups.Signals(3).Name = 'Signal 3'
      | sbobj.Groups.Signals(3).XData = [0 15 16 50]
      | sbobj.Groups.Signals(3).YData = [0 0 0 0]
      | sbobj.Groups.Signals(4).Name = 'Signal 4'
      | sbobj.Groups.Signals(4).XData = [0 12 12 13 13 50]
      | sbobj.Groups.Signals(4).YData = [0 0 1 1 0 0]
      | sbobj.Groups.Signals(5).Name = 'Signal 5'
      | sbobj.Groups.Signals(5).XData = [0 40 50]
      | sbobj.Groups.Signals(5).YData = [0 0 0]
      | sbobj.Groups.TimeRange = [0 50]
  Signal 1 : Outport  Tag=STV Outport
  Signal 2 : Outport  Tag=STV Outport  Port=2
  Signal 3 : Outport  Tag=STV Outport  Port=3
  Signal 4 : Outport  Tag=STV Outport  Port=4
  Signal 5 : Outport  Tag=STV Outport  Port=5
  wires:
  Demux/1 -> Signal 1/1
  FromWs/1 -> Demux/1
  Demux/2 -> Signal 2/1
  Demux/3 -> Signal 3/1
  Demux/4 -> Signal 4/1
  Demux/5 -> Signal 5/1

== system copy_final/PLANT/Live Request/Different TestCases/Signal Builder17 ==
  Demux : Demux  Tag=STV Demux  Outputs=5
  FromWs : FromWorkspace  Tag=STV FromWs  VariableName=tuvar  SampleTime=0
      SigBuilderData=|
      | common.afterFinalStr = 'Extrapolate'
      | common.sampleTime = 0
      | dataSet.timeRange = [0 120]
      | dataSet.name = 'Group 1'
      | sbobj.Groups.Name = 'Group 1'
      | sbobj.Groups.Signals(1).Name = 'Signal 1'
      | sbobj.Groups.Signals(1).XData = [0 10 10 11 11 120]
      | sbobj.Groups.Signals(1).YData = [0 0 1 1 -0.05 -0.05]
      | sbobj.Groups.Signals(2).Name = 'Signal 2'
      | sbobj.Groups.Signals(2).XData = [0 65 65 66 66 120]
      | sbobj.Groups.Signals(2).YData = [0 0 1 1 0 0]
      | sbobj.Groups.Signals(3).Name = 'Signal 3'
      | sbobj.Groups.Signals(3).XData = [0 80 80 81 81 120]
      | sbobj.Groups.Signals(3).YData = [0 0 1 1 0 0]
      | sbobj.Groups.Signals(4).Name = 'Signal 4'
      | sbobj.Groups.Signals(4).XData = [0 100 100 101 101 120]
      | sbobj.Groups.Signals(4).YData = [0 0 1 1 0 0]
      | sbobj.Groups.Signals(5).Name = 'Signal 5'
      | sbobj.Groups.Signals(5).XData = [0 40 120]
      | sbobj.Groups.Signals(5).YData = [0 0 0]
      | sbobj.Groups.TimeRange = [0 120]
  Signal 1 : Outport  Tag=STV Outport
  Signal 2 : Outport  Tag=STV Outport  Port=2
  Signal 3 : Outport  Tag=STV Outport  Port=3
  Signal 4 : Outport  Tag=STV Outport  Port=4
  Signal 5 : Outport  Tag=STV Outport  Port=5
  wires:
  Demux/1 -> Signal 1/1
  FromWs/1 -> Demux/1
  Demux/2 -> Signal 2/1
  Demux/3 -> Signal 3/1
  Demux/4 -> Signal 4/1
  Demux/5 -> Signal 5/1

== system copy_final/PLANT/Live Request/Different TestCases/Signal Builder18 ==
  Demux : Demux  Tag=STV Demux  Outputs=5
  FromWs : FromWorkspace  Tag=STV FromWs  VariableName=tuvar  SampleTime=0
      SigBuilderData=|
      | common.afterFinalStr = 'Extrapolate'
      | common.sampleTime = 0
      | dataSet.timeRange = [0 100]
      | dataSet.name = 'Group 1'
      | sbobj.Groups.Name = 'Group 1'
      | sbobj.Groups.Signals(1).Name = 'Signal 1'
      | sbobj.Groups.Signals(1).XData = [0 10 10 11 11 100]
      | sbobj.Groups.Signals(1).YData = [0 0 1 1 0 0]
      | sbobj.Groups.Signals(2).Name = 'Signal 2'
      | sbobj.Groups.Signals(2).XData = [0 40 40 41 41 100]
      | sbobj.Groups.Signals(2).YData = [0 0 1 1 0 0]
      | sbobj.Groups.Signals(3).Name = 'Signal 3'
      | sbobj.Groups.Signals(3).XData = [0 30 35 100]
      | sbobj.Groups.Signals(3).YData = [0 0 0 0]
      | sbobj.Groups.Signals(4).Name = 'Signal 4'
      | sbobj.Groups.Signals(4).XData = [0 20 22.6 100]
      | sbobj.Groups.Signals(4).YData = [0 0 0 0]
      | sbobj.Groups.Signals(5).Name = 'Signal 5'
      | sbobj.Groups.Signals(5).XData = [0 40 100]
      | sbobj.Groups.Signals(5).YData = [0 0 0]
      | sbobj.Groups.TimeRange = [0 100]
  Signal 1 : Outport  Tag=STV Outport
  Signal 2 : Outport  Tag=STV Outport  Port=2
  Signal 3 : Outport  Tag=STV Outport  Port=3
  Signal 4 : Outport  Tag=STV Outport  Port=4
  Signal 5 : Outport  Tag=STV Outport  Port=5
  wires:
  Demux/1 -> Signal 1/1
  FromWs/1 -> Demux/1
  Demux/2 -> Signal 2/1
  Demux/3 -> Signal 3/1
  Demux/4 -> Signal 4/1
  Demux/5 -> Signal 5/1

== system copy_final/PLANT/Live Request/Different TestCases/Signal Builder2 ==
  Demux : Demux  Tag=STV Demux  Outputs=5
  FromWs : FromWorkspace  Tag=STV FromWs  VariableName=tuvar  SampleTime=0
      SigBuilderData=|
      | common.afterFinalStr = 'Extrapolate'
      | common.sampleTime = 0
      | dataSet.timeRange = [0 50]
      | dataSet.name = 'Group 1'
      | sbobj.Groups.Name = 'Group 1'
      | sbobj.Groups.Signals(1).Name = 'Signal 1'
      | sbobj.Groups.Signals(1).XData = [0 4 6 50]
      | sbobj.Groups.Signals(1).YData = [0 0 0 0]
      | sbobj.Groups.Signals(2).Name = 'Signal 2'
      | sbobj.Groups.Signals(2).XData = [0 10 10 11 11 50]
      | sbobj.Groups.Signals(2).YData = [0 0 1 1 0 0]
      | sbobj.Groups.Signals(3).Name = 'Signal 3'
      | sbobj.Groups.Signals(3).XData = [0 21 30 50]
      | sbobj.Groups.Signals(3).YData = [0 0 0 0]
      | sbobj.Groups.Signals(4).Name = 'Signal 4'
      | sbobj.Groups.Signals(4).XData = [0 1 10 50]
      | sbobj.Groups.Signals(4).YData = [0 0 0 0]
      | sbobj.Groups.Signals(5).Name = 'Signal 5'
      | sbobj.Groups.Signals(5).XData = [0 40 50]
      | sbobj.Groups.Signals(5).YData = [0 0 0]
      | sbobj.Groups.TimeRange = [0 50]
  Signal 1 : Outport  Tag=STV Outport
  Signal 2 : Outport  Tag=STV Outport  Port=2
  Signal 3 : Outport  Tag=STV Outport  Port=3
  Signal 4 : Outport  Tag=STV Outport  Port=4
  Signal 5 : Outport  Tag=STV Outport  Port=5
  wires:
  Demux/1 -> Signal 1/1
  FromWs/1 -> Demux/1
  Demux/2 -> Signal 2/1
  Demux/3 -> Signal 3/1
  Demux/4 -> Signal 4/1
  Demux/5 -> Signal 5/1

== system copy_final/PLANT/Live Request/Different TestCases/Signal Builder3 ==
  Demux : Demux  Tag=STV Demux  Outputs=5
  FromWs : FromWorkspace  Tag=STV FromWs  VariableName=tuvar  SampleTime=0
      SigBuilderData=|
      | common.afterFinalStr = 'Extrapolate'
      | common.sampleTime = 0
      | dataSet.timeRange = [0 50]
      | dataSet.name = 'Group 1'
      | sbobj.Groups.Name = 'Group 1'
      | sbobj.Groups.Signals(1).Name = 'Signal 1'
      | sbobj.Groups.Signals(1).XData = [0 30 30 31 31 50]
      | sbobj.Groups.Signals(1).YData = [0 0 1 1 0 0]
      | sbobj.Groups.Signals(2).Name = 'Signal 2'
      | sbobj.Groups.Signals(2).XData = [0 20 20 21 21 50]
      | sbobj.Groups.Signals(2).YData = [0 0 1 1 0 0]
      | sbobj.Groups.Signals(3).Name = 'Signal 3'
      | sbobj.Groups.Signals(3).XData = [0 21 30 50]
      | sbobj.Groups.Signals(3).YData = [0 0 0 0]
      | sbobj.Groups.Signals(4).Name = 'Signal 4'
      | sbobj.Groups.Signals(4).XData = [0 1 10 50]
      | sbobj.Groups.Signals(4).YData = [0 0 0 0]
      | sbobj.Groups.Signals(5).Name = 'Signal 5'
      | sbobj.Groups.Signals(5).XData = [0 40 50]
      | sbobj.Groups.Signals(5).YData = [0 0 0]
      | sbobj.Groups.TimeRange = [0 50]
  Signal 1 : Outport  Tag=STV Outport
  Signal 2 : Outport  Tag=STV Outport  Port=2
  Signal 3 : Outport  Tag=STV Outport  Port=3
  Signal 4 : Outport  Tag=STV Outport  Port=4
  Signal 5 : Outport  Tag=STV Outport  Port=5
  wires:
  Demux/1 -> Signal 1/1
  FromWs/1 -> Demux/1
  Demux/2 -> Signal 2/1
  Demux/3 -> Signal 3/1
  Demux/4 -> Signal 4/1
  Demux/5 -> Signal 5/1

== system copy_final/PLANT/Live Request/Different TestCases/Signal Builder4 ==
  Demux : Demux  Tag=STV Demux  Outputs=5
  FromWs : FromWorkspace  Tag=STV FromWs  VariableName=tuvar  SampleTime=0
      SigBuilderData=|
      | common.afterFinalStr = 'Extrapolate'
      | common.sampleTime = 0
      | dataSet.timeRange = [0 50]
      | dataSet.name = 'Group 1'
      | sbobj.Groups.Name = 'Group 1'
      | sbobj.Groups.Signals(1).Name = 'Signal 1'
      | sbobj.Groups.Signals(1).XData = [0 20 20 21 21 50]
      | sbobj.Groups.Signals(1).YData = [0 0 1 1 0 0]
      | sbobj.Groups.Signals(2).Name = 'Signal 2'
      | sbobj.Groups.Signals(2).XData = [0 20 20 21 21 50]
      | sbobj.Groups.Signals(2).YData = [0 0 1 1 0 0]
      | sbobj.Groups.Signals(3).Name = 'Signal 3'
      | sbobj.Groups.Signals(3).XData = [0 21 30 50]
      | sbobj.Groups.Signals(3).YData = [0 0 0 0]
      | sbobj.Groups.Signals(4).Name = 'Signal 4'
      | sbobj.Groups.Signals(4).XData = [0 30 31 50]
      | sbobj.Groups.Signals(4).YData = [0 0 0 0]
      | sbobj.Groups.Signals(5).Name = 'Signal 5'
      | sbobj.Groups.Signals(5).XData = [0 40 50]
      | sbobj.Groups.Signals(5).YData = [0 0 0]
      | sbobj.Groups.TimeRange = [0 50]
  Signal 1 : Outport  Tag=STV Outport
  Signal 2 : Outport  Tag=STV Outport  Port=2
  Signal 3 : Outport  Tag=STV Outport  Port=3
  Signal 4 : Outport  Tag=STV Outport  Port=4
  Signal 5 : Outport  Tag=STV Outport  Port=5
  wires:
  Demux/1 -> Signal 1/1
  FromWs/1 -> Demux/1
  Demux/2 -> Signal 2/1
  Demux/3 -> Signal 3/1
  Demux/4 -> Signal 4/1
  Demux/5 -> Signal 5/1

== system copy_final/PLANT/Live Request/Different TestCases/Signal Builder5 ==
  Demux : Demux  Tag=STV Demux  Outputs=5
  FromWs : FromWorkspace  Tag=STV FromWs  VariableName=tuvar  SampleTime=0
      SigBuilderData=|
      | common.afterFinalStr = 'Extrapolate'
      | common.sampleTime = 0
      | dataSet.timeRange = [0 50]
      | dataSet.name = 'Group 1'
      | sbobj.Groups.Name = 'Group 1'
      | sbobj.Groups.Signals(1).Name = 'Signal 1'
      | sbobj.Groups.Signals(1).XData = [0 4 6 50]
      | sbobj.Groups.Signals(1).YData = [0 0 0 0]
      | sbobj.Groups.Signals(2).Name = 'Signal 2'
      | sbobj.Groups.Signals(2).XData = [0 10 10 11 11 50]
      | sbobj.Groups.Signals(2).YData = [0 0 1 1 0 0]
      | sbobj.Groups.Signals(3).Name = 'Signal 3'
      | sbobj.Groups.Signals(3).XData = [0 1 1 50]
      | sbobj.Groups.Signals(3).YData = [1 1 0 0]
      | sbobj.Groups.Signals(4).Name = 'Signal 4'
      | sbobj.Groups.Signals(4).XData = [0 5 6 50]
      | sbobj.Groups.Signals(4).YData = [0 0 0 0]
      | sbobj.Groups.Signals(5).Name = 'Signal 5'
      | sbobj.Groups.Signals(5).XData = [0 40 50]
      | sbobj.Groups.Signals(5).YData = [0 0 0]
      | sbobj.Groups.TimeRange = [0 50]
  Signal 1 : Outport  Tag=STV Outport
  Signal 2 : Outport  Tag=STV Outport  Port=2
  Signal 3 : Outport  Tag=STV Outport  Port=3
  Signal 4 : Outport  Tag=STV Outport  Port=4
  Signal 5 : Outport  Tag=STV Outport  Port=5
  wires:
  Demux/1 -> Signal 1/1
  FromWs/1 -> Demux/1
  Demux/2 -> Signal 2/1
  Demux/3 -> Signal 3/1
  Demux/4 -> Signal 4/1
  Demux/5 -> Signal 5/1

== system copy_final/PLANT/Live Request/Different TestCases/Signal Builder6 ==
  Demux : Demux  Tag=STV Demux  Outputs=5
  FromWs : FromWorkspace  Tag=STV FromWs  VariableName=tuvar  SampleTime=0
      SigBuilderData=|
      | common.afterFinalStr = 'Extrapolate'
      | common.sampleTime = 0
      | dataSet.timeRange = [0 50]
      | dataSet.name = 'Group 1'
      | sbobj.Groups.Name = 'Group 1'
      | sbobj.Groups.Signals(1).Name = 'Signal 1'
      | sbobj.Groups.Signals(1).XData = [0 40 40 41 41 50]
      | sbobj.Groups.Signals(1).YData = [0 0 1 1 0 0]
      | sbobj.Groups.Signals(2).Name = 'Signal 2'
      | sbobj.Groups.Signals(2).XData = [0 20 21 50]
      | sbobj.Groups.Signals(2).YData = [0 0 0 0]
      | sbobj.Groups.Signals(3).Name = 'Signal 3'
      | sbobj.Groups.Signals(3).XData = [0 21 30 50]
      | sbobj.Groups.Signals(3).YData = [0 0 0 0]
      | sbobj.Groups.Signals(4).Name = 'Signal 4'
      | sbobj.Groups.Signals(4).XData = [0 20 20 21 21 50]
      | sbobj.Groups.Signals(4).YData = [0 0 1 1 0 0]
      | sbobj.Groups.Signals(5).Name = 'Signal 5'
      | sbobj.Groups.Signals(5).XData = [0 40 50]
      | sbobj.Groups.Signals(5).YData = [0 0 0]
      | sbobj.Groups.TimeRange = [0 50]
  Signal 1 : Outport  Tag=STV Outport
  Signal 2 : Outport  Tag=STV Outport  Port=2
  Signal 3 : Outport  Tag=STV Outport  Port=3
  Signal 4 : Outport  Tag=STV Outport  Port=4
  Signal 5 : Outport  Tag=STV Outport  Port=5
  wires:
  Demux/1 -> Signal 1/1
  FromWs/1 -> Demux/1
  Demux/2 -> Signal 2/1
  Demux/3 -> Signal 3/1
  Demux/4 -> Signal 4/1
  Demux/5 -> Signal 5/1

== system copy_final/PLANT/Live Request/Different TestCases/Signal Builder7 ==
  Demux : Demux  Tag=STV Demux  Outputs=5
  FromWs : FromWorkspace  Tag=STV FromWs  VariableName=tuvar  SampleTime=0
      SigBuilderData=|
      | common.afterFinalStr = 'Extrapolate'
      | common.sampleTime = 0
      | dataSet.timeRange = [0 100]
      | dataSet.name = 'Group 1'
      | sbobj.Groups.Name = 'Group 1'
      | sbobj.Groups.Signals(1).Name = 'Signal 1'
      | sbobj.Groups.Signals(1).XData = [0 50 50 51 51 100]
      | sbobj.Groups.Signals(1).YData = [0 0 1 1 0 0]
      | sbobj.Groups.Signals(2).Name = 'Signal 2'
      | sbobj.Groups.Signals(2).XData = [0 40 40 41 41 100]
      | sbobj.Groups.Signals(2).YData = [0 0 1 1 0 0]
      | sbobj.Groups.Signals(3).Name = 'Signal 3'
      | sbobj.Groups.Signals(3).XData = [0 10 10 11 11 100]
      | sbobj.Groups.Signals(3).YData = [0 0 1 1 0 0]
      | sbobj.Groups.Signals(4).Name = 'Signal 4'
      | sbobj.Groups.Signals(4).XData = [0 20 21 100]
      | sbobj.Groups.Signals(4).YData = [0 0 0 0]
      | sbobj.Groups.Signals(5).Name = 'Signal 5'
      | sbobj.Groups.Signals(5).XData = [0 40 100]
      | sbobj.Groups.Signals(5).YData = [0 0 0]
      | sbobj.Groups.TimeRange = [0 100]
  Signal 1 : Outport  Tag=STV Outport
  Signal 2 : Outport  Tag=STV Outport  Port=2
  Signal 3 : Outport  Tag=STV Outport  Port=3
  Signal 4 : Outport  Tag=STV Outport  Port=4
  Signal 5 : Outport  Tag=STV Outport  Port=5
  wires:
  Demux/1 -> Signal 1/1
  FromWs/1 -> Demux/1
  Demux/2 -> Signal 2/1
  Demux/3 -> Signal 3/1
  Demux/4 -> Signal 4/1
  Demux/5 -> Signal 5/1
